simulink library "LibFactorGraph"  (Simulink 8.3)
settings: Solver=ode45  StartTime=0.0  StopTime=10.0  RelTol=1e-3
undefined symbols (not defined in the file or in its folder): bV, epsVal, eu, fcn, fP_0, fV, Hin_0, L_0, Nit_0, P_0, xi
libraries: LibFactorGraph x357
(part 2 of 4)

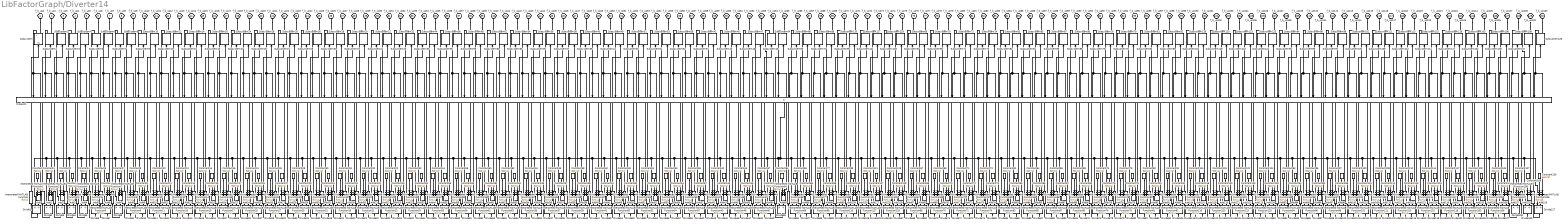
== system LibFactorGraph/Diverter14 ==
  Add{,1..129} (130 alike) : Sum
  Constant{,1..129} (130 alike) : Constant  Value=epsVal
  Divide{1..130} (130 alike) : Product  Inputs=*/
  Interpreted MATLAB Function{,1..129} (130 alike) : MATLABFcn  MATLABFcn=fcn(u)  Output1D=off
  Product1 : Product  Inputs=130  RndMeth=Zero
  Subsystem : Subsystem
  Subsystem{1..64,66..129} (128 alike) : LibFactorGraph/Diverter9/Subsystem
  Subsystem65 : LibFactorGraph/Diverter14/Subsystem
  f_b_up2 : PMIOPort  Port=1  Side=Left
  f_b_up1 : PMIOPort  Port=2  Side=Right
  f_b_up3 : PMIOPort  Port=3  Side=Left
  f_b_up4 : PMIOPort  Port=4  Side=Right
  f_b_up5 : PMIOPort  Port=5  Side=Left
  f_b_up6 : PMIOPort  Port=6  Side=Right
  f_b_up7 : PMIOPort  Port=7  Side=Left
  f_b_up8 : PMIOPort  Port=8  Side=Right
  f_b_up9 : PMIOPort  Port=9  Side=Left
  f_b_up10 : PMIOPort  Port=10  Side=Right
  f_b_up11 : PMIOPort  Port=11  Side=Left
  f_b_up12 : PMIOPort  Port=12  Side=Right
  f_b_up13 : PMIOPort  Port=13  Side=Left
  f_b_up14 : PMIOPort  Port=14  Side=Right
  f_b_up15 : PMIOPort  Port=15  Side=Left
  f_b_up16 : PMIOPort  Port=16  Side=Right
  f_b_up17 : PMIOPort  Port=17  Side=Left
  f_b_up18 : PMIOPort  Port=18  Side=Right
  f_b_up19 : PMIOPort  Port=19  Side=Left
  f_b_up20 : PMIOPort  Port=20  Side=Right
  f_b_up21 : PMIOPort  Port=21  Side=Left
  f_b_up22 : PMIOPort  Port=22  Side=Right
  f_b_up23 : PMIOPort  Port=23  Side=Left
  f_b_up24 : PMIOPort  Port=24  Side=Right
  f_b_up25 : PMIOPort  Port=25  Side=Left
  f_b_up26 : PMIOPort  Port=26  Side=Right
  f_b_up27 : PMIOPort  Port=27  Side=Left
  f_b_up28 : PMIOPort  Port=28  Side=Right
  f_b_up29 : PMIOPort  Port=29  Side=Left
  f_b_up30 : PMIOPort  Port=30  Side=Right
  f_b_up31 : PMIOPort  Port=31  Side=Left
  f_b_up32 : PMIOPort  Port=32  Side=Right
  f_b_up33 : PMIOPort  Port=33  Side=Left
  f_b_up34 : PMIOPort  Port=34  Side=Right
  f_b_up35 : PMIOPort  Port=35  Side=Left
  f_b_up36 : PMIOPort  Port=36  Side=Right
  f_b_up37 : PMIOPort  Port=37  Side=Left
  f_b_up38 : PMIOPort  Port=38  Side=Right
  f_b_up39 : PMIOPort  Port=39  Side=Left
  f_b_up40 : PMIOPort  Port=40  Side=Right
  f_b_up41 : PMIOPort  Port=41  Side=Left
  f_b_up42 : PMIOPort  Port=42  Side=Right
  f_b_up43 : PMIOPort  Port=43  Side=Left
  f_b_up44 : PMIOPort  Port=44  Side=Right
  f_b_up45 : PMIOPort  Port=45  Side=Left
  f_b_up46 : PMIOPort  Port=46  Side=Right
  f_b_up47 : PMIOPort  Port=47  Side=Left
  f_b_up48 : PMIOPort  Port=48  Side=Right
  f_b_up49 : PMIOPort  Port=49  Side=Left
  f_b_up50 : PMIOPort  Port=50  Side=Right
  f_b_up51 : PMIOPort  Port=51  Side=Left
  f_b_up52 : PMIOPort  Port=52  Side=Right
  f_b_up53 : PMIOPort  Port=53  Side=Left
  f_b_up54 : PMIOPort  Port=54  Side=Right
  f_b_up55 : PMIOPort  Port=55  Side=Left
  f_b_up56 : PMIOPort  Port=56  Side=Right
  f_b_up57 : PMIOPort  Port=57  Side=Left
  f_b_up58 : PMIOPort  Port=58  Side=Right
  f_b_up59 : PMIOPort  Port=59  Side=Left
  f_b_up60 : PMIOPort  Port=60  Side=Right
  f_b_up61 : PMIOPort  Port=61  Side=Left
  f_b_up62 : PMIOPort  Port=62  Side=Right
  f_b_up63 : PMIOPort  Port=63  Side=Left
  f_b_up64 : PMIOPort  Port=64  Side=Right
  f_b_up65 : PMIOPort  Port=65  Side=Left
  f_b_up66 : PMIOPort  Port=66  Side=Right
  f_b_up67 : PMIOPort  Port=67  Side=Left
  f_b_up68 : PMIOPort  Port=68  Side=Right
  f_b_up69 : PMIOPort  Port=69  Side=Left
  f_b_up70 : PMIOPort  Port=70  Side=Right
  f_b_up71 : PMIOPort  Port=71  Side=Left
  f_b_up72 : PMIOPort  Port=72  Side=Right
  f_b_up73 : PMIOPort  Port=73  Side=Left
  f_b_up74 : PMIOPort  Port=74  Side=Right
  f_b_up75 : PMIOPort  Port=75  Side=Left
  f_b_up76 : PMIOPort  Port=76  Side=Right
  f_b_up77 : PMIOPort  Port=77  Side=Left
  f_b_up78 : PMIOPort  Port=78  Side=Right
  f_b_up79 : PMIOPort  Port=79  Side=Left
  f_b_up80 : PMIOPort  Port=80  Side=Right
  f_b_up81 : PMIOPort  Port=81  Side=Left
  f_b_up82 : PMIOPort  Port=82  Side=Right
  f_b_up83 : PMIOPort  Port=83  Side=Left
  f_b_up84 : PMIOPort  Port=84  Side=Right
  f_b_up85 : PMIOPort  Port=85  Side=Left
  f_b_up86 : PMIOPort  Port=86  Side=Right
  f_b_up87 : PMIOPort  Port=87  Side=Left
  f_b_up88 : PMIOPort  Port=88  Side=Right
  f_b_up89 : PMIOPort  Port=89  Side=Left
  f_b_up90 : PMIOPort  Port=90  Side=Right
  f_b_up91 : PMIOPort  Port=91  Side=Left
  f_b_up92 : PMIOPort  Port=92  Side=Right
  f_b_up93 : PMIOPort  Port=93  Side=Left
  f_b_up94 : PMIOPort  Port=94  Side=Right
  f_b_up95 : PMIOPort  Port=95  Side=Left
  f_b_up96 : PMIOPort  Port=96  Side=Right
  f_b_up97 : PMIOPort  Port=97  Side=Left
  f_b_up98 : PMIOPort  Port=98  Side=Right
  f_b_up99 : PMIOPort  Port=99  Side=Left
  f_b_up100 : PMIOPort  Port=100  Side=Right
  f_b_up101 : PMIOPort  Port=101  Side=Left
  f_b_up102 : PMIOPort  Port=102  Side=Right
  f_b_up103 : PMIOPort  Port=103  Side=Left
  f_b_up104 : PMIOPort  Port=104  Side=Right
  f_b_up105 : PMIOPort  Port=105  Side=Left
  f_b_up106 : PMIOPort  Port=106  Side=Right
  f_b_up107 : PMIOPort  Port=107  Side=Left
  f_b_up108 : PMIOPort  Port=108  Side=Right
  f_b_up109 : PMIOPort  Port=109  Side=Left
  f_b_up110 : PMIOPort  Port=110  Side=Right
  f_b_up111 : PMIOPort  Port=111  Side=Left
  f_b_up112 : PMIOPort  Port=112  Side=Right
  f_b_up113 : PMIOPort  Port=113  Side=Left
  f_b_up114 : PMIOPort  Port=114  Side=Right
  f_b_up115 : PMIOPort  Port=115  Side=Left
  f_b_up116 : PMIOPort  Port=116  Side=Right
  f_b_up117 : PMIOPort  Port=117  Side=Left
  f_b_up118 : PMIOPort  Port=118  Side=Right
  f_b_up119 : PMIOPort  Port=119  Side=Left
  f_b_up120 : PMIOPort  Port=120  Side=Right
  f_b_up121 : PMIOPort  Port=121  Side=Left
  f_b_up122 : PMIOPort  Port=122  Side=Right
  f_b_up123 : PMIOPort  Port=123  Side=Left
  f_b_up124 : PMIOPort  Port=124  Side=Right
  f_b_up125 : PMIOPort  Port=125  Side=Left
  f_b_up126 : PMIOPort  Port=126  Side=Right
  f_b_up127 : PMIOPort  Port=127  Side=Left
  f_b_up128 : PMIOPort  Port=128  Side=Right
  f_b_up129 : PMIOPort  Port=129  Side=Left
  f_b_up130 : PMIOPort  Port=130  Side=Right
  wires:
  Constant/1 -> Add/1
  Interpreted MATLAB Function/1 -> Subsystem/1(In1)
  Subsystem/1(Out1) -> Product1/1, Add/2
  Divide1/1 -> Interpreted MATLAB Function/1
  Constant1/1 -> Add1/1
  Interpreted MATLAB Function1/1 -> Subsystem1/1
  Subsystem1/1 -> Product1/2, Add1/2
  Divide2/1 -> Interpreted MATLAB Function1/1
  Constant2/1 -> Add2/1
  Interpreted MATLAB Function2/1 -> Subsystem2/1
  Subsystem2/1 -> Product1/3, Add2/2
  Divide3/1 -> Interpreted MATLAB Function2/1
  Constant3/1 -> Add3/1
  Interpreted MATLAB Function3/1 -> Subsystem3/1
  Subsystem3/1 -> Product1/4, Add3/2
  Divide4/1 -> Interpreted MATLAB Function3/1
  Constant4/1 -> Add4/1
  Interpreted MATLAB Function4/1 -> Subsystem4/1
  Subsystem4/1 -> Product1/5, Add4/2
  Divide5/1 -> Interpreted MATLAB Function4/1
  Constant5/1 -> Add5/1
  Interpreted MATLAB Function5/1 -> Subsystem5/1
  Subsystem5/1 -> Product1/6, Add5/2
  Divide6/1 -> Interpreted MATLAB Function5/1
  Constant6/1 -> Add6/1
  Interpreted MATLAB Function6/1 -> Subsystem6/1
  Subsystem6/1 -> Product1/7, Add6/2
  Divide7/1 -> Interpreted MATLAB Function6/1
  Constant7/1 -> Add7/1
  Interpreted MATLAB Function7/1 -> Subsystem7/1
  Subsystem7/1 -> Product1/8, Add7/2
  Divide8/1 -> Interpreted MATLAB Function7/1
  Add/1 -> Divide1/2
  Add1/1 -> Divide2/2
  Add2/1 -> Divide3/2
  Add3/1 -> Divide4/2
  Add4/1 -> Divide5/2
  Add5/1 -> Divide6/2
  Add6/1 -> Divide7/2
  Add7/1 -> Divide8/2
  Constant8/1 -> Add8/1
  Interpreted MATLAB Function8/1 -> Subsystem8/1
  Subsystem8/1 -> Product1/9, Add8/2
  Divide9/1 -> Interpreted MATLAB Function8/1
  Constant9/1 -> Add9/1
  Interpreted MATLAB Function9/1 -> Subsystem9/1
  Subsystem9/1 -> Product1/10, Add9/2
  Divide10/1 -> Interpreted MATLAB Function9/1
  Constant10/1 -> Add10/1
  Interpreted MATLAB Function10/1 -> Subsystem10/1
  Subsystem10/1 -> Product1/11, Add10/2
  Divide11/1 -> Interpreted MATLAB Function10/1
  Constant11/1 -> Add11/1
  Interpreted MATLAB Function11/1 -> Subsystem11/1
  Subsystem11/1 -> Product1/12, Add11/2
  Divide12/1 -> Interpreted MATLAB Function11/1
  Constant12/1 -> Add12/1
  Interpreted MATLAB Function12/1 -> Subsystem12/1
  Subsystem12/1 -> Product1/13, Add12/2
  Divide13/1 -> Interpreted MATLAB Function12/1
  Constant13/1 -> Add13/1
  Interpreted MATLAB Function13/1 -> Subsystem13/1
  Subsystem13/1 -> Product1/14, Add13/2
  Divide14/1 -> Interpreted MATLAB Function13/1
  Constant14/1 -> Add14/1
  Interpreted MATLAB Function14/1 -> Subsystem14/1
  Subsystem14/1 -> Product1/15, Add14/2
  Divide15/1 -> Interpreted MATLAB Function14/1
  Constant15/1 -> Add15/1
  Interpreted MATLAB Function15/1 -> Subsystem15/1
  Subsystem15/1 -> Product1/16, Add15/2
  Divide16/1 -> Interpreted MATLAB Function15/1
  Add8/1 -> Divide9/2
  Add9/1 -> Divide10/2
  Add10/1 -> Divide11/2
  Add11/1 -> Divide12/2
  Add12/1 -> Divide13/2
  Add13/1 -> Divide14/2
  Add14/1 -> Divide15/2
  Add15/1 -> Divide16/2
  Constant16/1 -> Add16/1
  Interpreted MATLAB Function16/1 -> Subsystem16/1
  Subsystem16/1 -> Product1/17, Add16/2
  Divide17/1 -> Interpreted MATLAB Function16/1
  Constant17/1 -> Add17/1
  Interpreted MATLAB Function17/1 -> Subsystem17/1
  Subsystem17/1 -> Product1/18, Add17/2
  Divide25/1 -> Interpreted MATLAB Function17/1
  Constant24/1 -> Add24/1
  Interpreted MATLAB Function24/1 -> Subsystem24/1
  Subsystem24/1 -> Product1/19, Add24/2
  Divide26/1 -> Interpreted MATLAB Function24/1
  Constant25/1 -> Add25/1
  Interpreted MATLAB Function25/1 -> Subsystem25/1
  Subsystem25/1 -> Product1/20, Add25/2
  Divide27/1 -> Interpreted MATLAB Function25/1
  Constant26/1 -> Add26/1
  Interpreted MATLAB Function26/1 -> Subsystem26/1
  Subsystem26/1 -> Product1/21, Add26/2
  Divide28/1 -> Interpreted MATLAB Function26/1
  Constant27/1 -> Add27/1
  Interpreted MATLAB Function27/1 -> Subsystem27/1
  Subsystem27/1 -> Product1/22, Add27/2
  Divide29/1 -> Interpreted MATLAB Function27/1
  Constant28/1 -> Add28/1
  Interpreted MATLAB Function28/1 -> Subsystem28/1
  Subsystem28/1 -> Product1/23, Add28/2
  Divide30/1 -> Interpreted MATLAB Function28/1
  Constant29/1 -> Add29/1
  Interpreted MATLAB Function29/1 -> Subsystem29/1
  Subsystem29/1 -> Product1/24, Add29/2
  Divide31/1 -> Interpreted MATLAB Function29/1
  Add16/1 -> Divide17/2
  Add17/1 -> Divide25/2
  Add24/1 -> Divide26/2
  Add25/1 -> Divide27/2
  Add26/1 -> Divide28/2
  Add27/1 -> Divide29/2
  Add28/1 -> Divide30/2
  Add29/1 -> Divide31/2
  Constant30/1 -> Add30/1
  Interpreted MATLAB Function30/1 -> Subsystem30/1
  Subsystem30/1 -> Product1/25, Add30/2
  Divide32/1 -> Interpreted MATLAB Function30/1
  Constant31/1 -> Add31/1
  Interpreted MATLAB Function31/1 -> Subsystem31/1
  Subsystem31/1 -> Product1/26, Add31/2
  Divide18/1 -> Interpreted MATLAB Function31/1
  Constant18/1 -> Add18/1
  Interpreted MATLAB Function18/1 -> Subsystem18/1
  Subsystem18/1 -> Product1/27, Add18/2
  Divide19/1 -> Interpreted MATLAB Function18/1
  Constant19/1 -> Add19/1
  Interpreted MATLAB Function19/1 -> Subsystem19/1
  Subsystem19/1 -> Product1/28, Add19/2
  Divide20/1 -> Interpreted MATLAB Function19/1
  Constant20/1 -> Add20/1
  Interpreted MATLAB Function20/1 -> Subsystem20/1
  Subsystem20/1 -> Product1/29, Add20/2
  Divide21/1 -> Interpreted MATLAB Function20/1
  Constant21/1 -> Add21/1
  Interpreted MATLAB Function21/1 -> Subsystem21/1
  Subsystem21/1 -> Product1/30, Add21/2
  Divide22/1 -> Interpreted MATLAB Function21/1
  Constant22/1 -> Add22/1
  Interpreted MATLAB Function22/1 -> Subsystem22/1
  Subsystem22/1 -> Product1/31, Add22/2
  Divide23/1 -> Interpreted MATLAB Function22/1
  Constant23/1 -> Add23/1
  Interpreted MATLAB Function23/1 -> Subsystem23/1
  Subsystem23/1 -> Product1/32, Add23/2
  Divide24/1 -> Interpreted MATLAB Function23/1
  Add30/1 -> Divide32/2
  Add31/1 -> Divide18/2
  Add18/1 -> Divide19/2
  Add19/1 -> Divide20/2
  Add20/1 -> Divide21/2
  Add21/1 -> Divide22/2
  Add22/1 -> Divide23/2
  Add23/1 -> Divide24/2
  Constant32/1 -> Add32/1
  Interpreted MATLAB Function32/1 -> Subsystem32/1
  Subsystem32/1 -> Product1/33, Add32/2
  Divide33/1 -> Interpreted MATLAB Function32/1
  Constant33/1 -> Add33/1
  Interpreted MATLAB Function33/1 -> Subsystem33/1
  Subsystem33/1 -> Product1/34, Add33/2
  Divide44/1 -> Interpreted MATLAB Function33/1
  Constant44/1 -> Add44/1
  Interpreted MATLAB Function44/1 -> Subsystem44/1
  Subsystem44/1 -> Product1/35, Add44/2
  Divide55/1 -> Interpreted MATLAB Function44/1
  Constant55/1 -> Add55/1
  Interpreted MATLAB Function55/1 -> Subsystem55/1
  Subsystem55/1 -> Product1/36, Add55/2
  Divide59/1 -> Interpreted MATLAB Function55/1
  Constant58/1 -> Add58/1
  Interpreted MATLAB Function58/1 -> Subsystem58/1
  Subsystem58/1 -> Product1/37, Add58/2
  Divide60/1 -> Interpreted MATLAB Function58/1
  Constant59/1 -> Add59/1
  Interpreted MATLAB Function59/1 -> Subsystem59/1
  Subsystem59/1 -> Product1/38, Add59/2
  Divide61/1 -> Interpreted MATLAB Function59/1
  Constant60/1 -> Add60/1
  Interpreted MATLAB Function60/1 -> Subsystem60/1
  Subsystem60/1 -> Product1/39, Add60/2
  Divide62/1 -> Interpreted MATLAB Function60/1
  Constant61/1 -> Add61/1
  Interpreted MATLAB Function61/1 -> Subsystem61/1
  Subsystem61/1 -> Product1/40, Add61/2
  Divide63/1 -> Interpreted MATLAB Function61/1
  Add32/1 -> Divide33/2
  Add33/1 -> Divide44/2
  Add44/1 -> Divide55/2
  Add55/1 -> Divide59/2
  Add58/1 -> Divide60/2
  Add59/1 -> Divide61/2
  Add60/1 -> Divide62/2
  Add61/1 -> Divide63/2
  Constant62/1 -> Add62/1
  Interpreted MATLAB Function62/1 -> Subsystem62/1
  Subsystem62/1 -> Product1/41, Add62/2
  Divide64/1 -> Interpreted MATLAB Function62/1
  Constant63/1 -> Add63/1
  Interpreted MATLAB Function63/1 -> Subsystem63/1
  Subsystem63/1 -> Product1/42, Add63/2
  Divide34/1 -> Interpreted MATLAB Function63/1
  Constant34/1 -> Add34/1
  Interpreted MATLAB Function34/1 -> Subsystem34/1
  Subsystem34/1 -> Product1/43, Add34/2
  Divide35/1 -> Interpreted MATLAB Function34/1
  Constant35/1 -> Add35/1
  Interpreted MATLAB Function35/1 -> Subsystem35/1
  Subsystem35/1 -> Product1/44, Add35/2
  Divide36/1 -> Interpreted MATLAB Function35/1
  Constant36/1 -> Add36/1
  Interpreted MATLAB Function36/1 -> Subsystem36/1
  Subsystem36/1 -> Product1/45, Add36/2
  Divide37/1 -> Interpreted MATLAB Function36/1
  Constant37/1 -> Add37/1
  Interpreted MATLAB Function37/1 -> Subsystem37/1
  Subsystem37/1 -> Product1/46, Add37/2
  Divide38/1 -> Interpreted MATLAB Function37/1
  Constant38/1 -> Add38/1
  Interpreted MATLAB Function38/1 -> Subsystem38/1
  Subsystem38/1 -> Product1/47, Add38/2
  Divide39/1 -> Interpreted MATLAB Function38/1
  Constant39/1 -> Add39/1
  Interpreted MATLAB Function39/1 -> Subsystem39/1
  Subsystem39/1 -> Product1/48, Add39/2
  Divide40/1 -> Interpreted MATLAB Function39/1
  Add62/1 -> Divide64/2
  Add63/1 -> Divide34/2
  Add34/1 -> Divide35/2
  Add35/1 -> Divide36/2
  Add36/1 -> Divide37/2
  Add37/1 -> Divide38/2
  Add38/1 -> Divide39/2
  Add39/1 -> Divide40/2
  Constant40/1 -> Add40/1
  Interpreted MATLAB Function40/1 -> Subsystem40/1
  Subsystem40/1 -> Product1/49, Add40/2
  Divide41/1 -> Interpreted MATLAB Function40/1
  Constant41/1 -> Add41/1
  Interpreted MATLAB Function41/1 -> Subsystem41/1
  Subsystem41/1 -> Product1/50, Add41/2
  Divide50/1 -> Interpreted MATLAB Function41/1
  Constant49/1 -> Add49/1
  Interpreted MATLAB Function49/1 -> Subsystem49/1
  Subsystem49/1 -> Product1/51, Add49/2
  Divide51/1 -> Interpreted MATLAB Function49/1
  Constant50/1 -> Add50/1
  Interpreted MATLAB Function50/1 -> Subsystem50/1
  Subsystem50/1 -> Product1/52, Add50/2
  Divide52/1 -> Interpreted MATLAB Function50/1
  Constant51/1 -> Add51/1
  Interpreted MATLAB Function51/1 -> Subsystem51/1
  Subsystem51/1 -> Product1/53, Add51/2
  Divide53/1 -> Interpreted MATLAB Function51/1
  Constant52/1 -> Add52/1
  Interpreted MATLAB Function52/1 -> Subsystem52/1
  Subsystem52/1 -> Product1/54, Add52/2
  Divide54/1 -> Interpreted MATLAB Function52/1
  Constant53/1 -> Add53/1
  Interpreted MATLAB Function53/1 -> Subsystem53/1
  Subsystem53/1 -> Product1/55, Add53/2
  Divide56/1 -> Interpreted MATLAB Function53/1
  Constant54/1 -> Add54/1
  Interpreted MATLAB Function54/1 -> Subsystem54/1
  Subsystem54/1 -> Product1/56, Add54/2
  Divide57/1 -> Interpreted MATLAB Function54/1
  Add40/1 -> Divide41/2
  Add41/1 -> Divide50/2
  Add49/1 -> Divide51/2
  Add50/1 -> Divide52/2
  Add51/1 -> Divide53/2
  Add52/1 -> Divide54/2
  Add53/1 -> Divide56/2
  Add54/1 -> Divide57/2
  Constant56/1 -> Add56/1
  Interpreted MATLAB Function56/1 -> Subsystem56/1
  Subsystem56/1 -> Product1/57, Add56/2
  Divide58/1 -> Interpreted MATLAB Function56/1
  Constant57/1 -> Add57/1
  Interpreted MATLAB Function57/1 -> Subsystem57/1
  Subsystem57/1 -> Product1/58, Add57/2
  Divide42/1 -> Interpreted MATLAB Function57/1
  Constant42/1 -> Add42/1
  Interpreted MATLAB Function42/1 -> Subsystem42/1
  Subsystem42/1 -> Product1/59, Add42/2
  Divide43/1 -> Interpreted MATLAB Function42/1
  Constant43/1 -> Add43/1
  Interpreted MATLAB Function43/1 -> Subsystem43/1
  Subsystem43/1 -> Product1/60, Add43/2
  Divide45/1 -> Interpreted MATLAB Function43/1
  Constant45/1 -> Add45/1
  Interpreted MATLAB Function45/1 -> Subsystem45/1
  Subsystem45/1 -> Product1/61, Add45/2
  Divide46/1 -> Interpreted MATLAB Function45/1
  Constant46/1 -> Add46/1
  Interpreted MATLAB Function46/1 -> Subsystem46/1
  Subsystem46/1 -> Product1/62, Add46/2
  Divide47/1 -> Interpreted MATLAB Function46/1
  Constant47/1 -> Add47/1
  Interpreted MATLAB Function47/1 -> Subsystem47/1
  Subsystem47/1 -> Product1/63, Add47/2
  Divide48/1 -> Interpreted MATLAB Function47/1
  Interpreted MATLAB Function48/1 -> Subsystem48/1
  Subsystem48/1 -> Product1/64, Add64/2
  Divide49/1 -> Interpreted MATLAB Function48/1
  Add56/1 -> Divide58/2
  Add57/1 -> Divide42/2
  Add42/1 -> Divide43/2
  Add43/1 -> Divide45/2
  Add45/1 -> Divide46/2
  Add46/1 -> Divide47/2
  Add47/1 -> Divide48/2
  Add64/1 -> Divide49/2
  Constant64/1 -> Add65/1
  Interpreted MATLAB Function64/1 -> Subsystem64/1
  Subsystem64/1 -> Product1/65, Add65/2
  Divide65/1 -> Interpreted MATLAB Function64/1
  Add65/1 -> Divide65/2
  Constant48/1 -> Add64/1
  Constant65/1 -> Add48/1
  Interpreted MATLAB Function65/1 -> Subsystem65/1
  Subsystem65/1 -> Product1/66, Add48/2
  Divide66/1 -> Interpreted MATLAB Function65/1
  Product1/1 -> Divide127/1, Divide109/1, Divide108/1, Divide107/1, Divide106/1, Divide105/1, Divide103/1, Divide102/1, Divide119/1, Divide118/1, Divide117/1, Divide115/1, Divide114/1, Divide113/1, Divide112/1, Divide111/1, Divide101/1, Divide100/1, Divide98/1, Divide97/1, Divide96/1, Divide95/1, Divide94/1, Divide93/1, Divide126/1, Divide125/1, Divide124/1, Divide123/1, Divide122/1, Divide120/1, Divide116/1, Divide104/1, Divide92/1, Divide82/1, Divide81/1, Divide80/1, Divide79/1, Divide78/1, Divide76/1, Divide75/1, Divide91/1, Divide90/1, Divide89/1, Divide87/1, Divide86/1, Divide85/1, Divide84/1, Divide83/1, Divide74/1, Divide73/1, Divide72/1, Divide71/1, Divide70/1, Divide69/1, Divide68/1, Divide67/1, Divide130/1, Divide129/1, Divide128/1, Divide121/1, Divide110/1, Divide99/1, Divide88/1, Divide77/1, Divide66/1, Divide33/1, Divide24/1, Divide23/1, Divide22/1, Divide20/1, Divide19/1, Divide18/1, Divide32/1, Divide31/1, Divide30/1, Divide29/1, Divide28/1, Divide27/1, Divide26/1, Divide25/1, Divide17/1, Divide14/1, Divide13/1, Divide12/1, Divide10/1, Divide9/1, Divide8/1, Divide7/1, Divide6/1, Divide5/1, Divide4/1, Divide3/1, Divide2/1, Divide1/1, Divide11/1, Divide15/1, Divide16/1, Divide21/1, Divide44/1, Divide55/1, Divide59/1, Divide60/1, Divide61/1, Divide62/1, Divide63/1, Divide64/1, Divide34/1, Divide35/1, Divide36/1, Divide37/1, Divide38/1, Divide39/1, Divide40/1, Divide41/1, Divide50/1, Divide51/1, Divide52/1, Divide53/1, Divide54/1, Divide56/1, Divide57/1, Divide58/1, Divide42/1, Divide43/1, Divide45/1, Divide46/1, Divide47/1, Divide48/1, Divide49/1, Divide65/1
  Constant66/1 -> Add66/1
  Interpreted MATLAB Function66/1 -> Subsystem66/1
  Subsystem66/1 -> Product1/67, Add66/2
  Divide77/1 -> Interpreted MATLAB Function66/1
  Constant77/1 -> Add77/1
  Interpreted MATLAB Function77/1 -> Subsystem77/1
  Subsystem77/1 -> Product1/68, Add77/2
  Divide88/1 -> Interpreted MATLAB Function77/1
  Constant88/1 -> Add88/1
  Interpreted MATLAB Function88/1 -> Subsystem88/1
  Subsystem88/1 -> Product1/69, Add88/2
  Divide99/1 -> Interpreted MATLAB Function88/1
  Constant99/1 -> Add99/1
  Interpreted MATLAB Function99/1 -> Subsystem99/1
  Subsystem99/1 -> Product1/70, Add99/2
  Divide110/1 -> Interpreted MATLAB Function99/1
  Constant110/1 -> Add109/1
  Interpreted MATLAB Function110/1 -> Subsystem110/1
  Subsystem110/1 -> Product1/71, Add109/2
  Divide121/1 -> Interpreted MATLAB Function110/1
  Constant121/1 -> Add120/1
  Interpreted MATLAB Function121/1 -> Subsystem121/1
  Subsystem121/1 -> Product1/72, Add120/2
  Divide128/1 -> Interpreted MATLAB Function121/1
  Constant127/1 -> Add127/1
  Interpreted MATLAB Function127/1 -> Subsystem127/1
  Subsystem127/1 -> Product1/73, Add127/2
  Divide129/1 -> Interpreted MATLAB Function127/1
  Add48/1 -> Divide66/2
  Add66/1 -> Divide77/2
  Add77/1 -> Divide88/2
  Add88/1 -> Divide99/2
  Add99/1 -> Divide110/2
  Add109/1 -> Divide121/2
  Add120/1 -> Divide128/2
  Add127/1 -> Divide129/2
  Constant128/1 -> Add128/1
  Interpreted MATLAB Function128/1 -> Subsystem128/1
  Subsystem128/1 -> Product1/74, Add128/2
  Divide130/1 -> Interpreted MATLAB Function128/1
  Constant129/1 -> Add129/1
  Interpreted MATLAB Function129/1 -> Subsystem129/1
  Subsystem129/1 -> Product1/75, Add129/2
  Divide67/1 -> Interpreted MATLAB Function129/1
  Constant67/1 -> Add67/1
  Interpreted MATLAB Function67/1 -> Subsystem67/1
  Subsystem67/1 -> Product1/76, Add67/2
  Divide68/1 -> Interpreted MATLAB Function67/1
  Constant68/1 -> Add68/1
  Interpreted MATLAB Function68/1 -> Subsystem68/1
  Subsystem68/1 -> Product1/77, Add68/2
  Divide69/1 -> Interpreted MATLAB Function68/1
  Constant69/1 -> Add69/1
  Interpreted MATLAB Function69/1 -> Subsystem69/1
  Subsystem69/1 -> Product1/78, Add69/2
  Divide70/1 -> Interpreted MATLAB Function69/1
  Constant70/1 -> Add70/1
  Interpreted MATLAB Function70/1 -> Subsystem70/1
  Subsystem70/1 -> Product1/79, Add70/2
  Divide71/1 -> Interpreted MATLAB Function70/1
  Constant71/1 -> Add71/1
  Interpreted MATLAB Function71/1 -> Subsystem71/1
  Subsystem71/1 -> Product1/80, Add71/2
  Divide72/1 -> Interpreted MATLAB Function71/1
  Constant72/1 -> Add72/1
  Interpreted MATLAB Function72/1 -> Subsystem72/1
  Subsystem72/1 -> Product1/81, Add72/2
  Divide73/1 -> Interpreted MATLAB Function72/1
  Add128/1 -> Divide130/2
  Add129/1 -> Divide67/2
  Add67/1 -> Divide68/2
  Add68/1 -> Divide69/2
  Add69/1 -> Divide70/2
  Add70/1 -> Divide71/2
  Add71/1 -> Divide72/2
  Add72/1 -> Divide73/2
  Constant73/1 -> Add73/1
  Interpreted MATLAB Function73/1 -> Subsystem73/1
  Subsystem73/1 -> Product1/82, Add73/2
  Divide74/1 -> Interpreted MATLAB Function73/1
  Constant74/1 -> Add74/1
  Interpreted MATLAB Function74/1 -> Subsystem74/1
  Subsystem74/1 -> Product1/83, Add74/2
  Divide83/1 -> Interpreted MATLAB Function74/1
  Constant82/1 -> Add82/1
  Interpreted MATLAB Function82/1 -> Subsystem82/1
  Subsystem82/1 -> Product1/84, Add82/2
  Divide84/1 -> Interpreted MATLAB Function82/1
  Constant83/1 -> Add83/1
  Interpreted MATLAB Function83/1 -> Subsystem83/1
  Subsystem83/1 -> Product1/85, Add83/2
  Divide85/1 -> Interpreted MATLAB Function83/1
  Constant84/1 -> Add84/1
  Interpreted MATLAB Function84/1 -> Subsystem84/1
  Subsystem84/1 -> Product1/86, Add84/2
  Divide86/1 -> Interpreted MATLAB Function84/1
  Constant85/1 -> Add85/1
  Interpreted MATLAB Function85/1 -> Subsystem85/1
  Subsystem85/1 -> Product1/87, Add85/2
  Divide87/1 -> Interpreted MATLAB Function85/1
  Constant86/1 -> Add86/1
  Interpreted MATLAB Function86/1 -> Subsystem86/1
  Subsystem86/1 -> Product1/88, Add86/2
  Divide89/1 -> Interpreted MATLAB Function86/1
  Constant87/1 -> Add87/1
  Interpreted MATLAB Function87/1 -> Subsystem87/1
  Subsystem87/1 -> Product1/89, Add87/2
  Divide90/1 -> Interpreted MATLAB Function87/1
  Add73/1 -> Divide74/2
  Add74/1 -> Divide83/2
  Add82/1 -> Divide84/2
  Add83/1 -> Divide85/2
  Add84/1 -> Divide86/2
  Add85/1 -> Divide87/2
  Add86/1 -> Divide89/2
  Add87/1 -> Divide90/2
  Constant89/1 -> Add89/1
  Interpreted MATLAB Function89/1 -> Subsystem89/1
  Subsystem89/1 -> Product1/90, Add89/2
  Divide91/1 -> Interpreted MATLAB Function89/1
  Constant90/1 -> Add90/1
  Interpreted MATLAB Function90/1 -> Subsystem90/1
  Subsystem90/1 -> Product1/91, Add90/2
  Divide75/1 -> Interpreted MATLAB Function90/1
  Constant75/1 -> Add75/1
  Interpreted MATLAB Function75/1 -> Subsystem75/1
  Subsystem75/1 -> Product1/92, Add75/2
  Divide76/1 -> Interpreted MATLAB Function75/1
  Constant76/1 -> Add76/1
  Interpreted MATLAB Function76/1 -> Subsystem76/1
  Subsystem76/1 -> Product1/93, Add76/2
  Divide78/1 -> Interpreted MATLAB Function76/1
  Constant78/1 -> Add78/1
  Interpreted MATLAB Function78/1 -> Subsystem78/1
  Subsystem78/1 -> Product1/94, Add78/2
  Divide79/1 -> Interpreted MATLAB Function78/1
  Constant79/1 -> Add79/1
  Interpreted MATLAB Function79/1 -> Subsystem79/1
  Subsystem79/1 -> Product1/95, Add79/2
  Divide80/1 -> Interpreted MATLAB Function79/1
  Constant80/1 -> Add80/1
  Interpreted MATLAB Function80/1 -> Subsystem80/1
  Subsystem80/1 -> Product1/96, Add80/2
  Divide81/1 -> Interpreted MATLAB Function80/1
  Constant81/1 -> Add81/1
  Interpreted MATLAB Function81/1 -> Subsystem81/1
  Subsystem81/1 -> Product1/97, Add81/2
  Divide82/1 -> Interpreted MATLAB Function81/1
  Add89/1 -> Divide91/2
  Add90/1 -> Divide75/2
  Add75/1 -> Divide76/2
  Add76/1 -> Divide78/2
  Add78/1 -> Divide79/2
  Add79/1 -> Divide80/2
  Add80/1 -> Divide81/2
  Add81/1 -> Divide82/2
  Constant91/1 -> Add91/1
  Interpreted MATLAB Function91/1 -> Subsystem91/1
  Subsystem91/1 -> Product1/98, Add91/2
  Divide92/1 -> Interpreted MATLAB Function91/1
  Constant92/1 -> Add92/1
  Interpreted MATLAB Function92/1 -> Subsystem92/1
  Subsystem92/1 -> Product1/99, Add92/2
  Divide104/1 -> Interpreted MATLAB Function92/1
  Constant104/1 -> Add104/1
  Interpreted MATLAB Function104/1 -> Subsystem104/1
  Subsystem104/1 -> Product1/100, Add104/2
  Divide116/1 -> Interpreted MATLAB Function104/1
  Constant116/1 -> Add115/1
  Interpreted MATLAB Function116/1 -> Subsystem116/1
  Subsystem116/1 -> Product1/101, Add115/2
  Divide120/1 -> Interpreted MATLAB Function116/1
  Constant119/1 -> Add118/1
  Interpreted MATLAB Function119/1 -> Subsystem119/1
  Subsystem119/1 -> Product1/102, Add118/2
  Divide122/1 -> Interpreted MATLAB Function119/1
  Constant120/1 -> Add119/1
  Interpreted MATLAB Function120/1 -> Subsystem120/1
  Subsystem120/1 -> Product1/103, Add119/2
  Divide123/1 -> Interpreted MATLAB Function120/1
  Constant122/1 -> Add121/1
  Interpreted MATLAB Function122/1 -> Subsystem122/1
  Subsystem122/1 -> Product1/104, Add121/2
  Divide124/1 -> Interpreted MATLAB Function122/1
  Constant123/1 -> Add122/1
  Interpreted MATLAB Function123/1 -> Subsystem123/1
  Subsystem123/1 -> Product1/105, Add122/2
  Divide125/1 -> Interpreted MATLAB Function123/1
  Add91/1 -> Divide92/2
  Add92/1 -> Divide104/2
  Add104/1 -> Divide116/2
  Add115/1 -> Divide120/2
  Add118/1 -> Divide122/2
  Add119/1 -> Divide123/2
  Add121/1 -> Divide124/2
  Add122/1 -> Divide125/2
  Constant124/1 -> Add123/1
  Interpreted MATLAB Function124/1 -> Subsystem124/1
  Subsystem124/1 -> Product1/106, Add123/2
  Divide126/1 -> Interpreted MATLAB Function124/1
  Constant125/1 -> Add124/1
  Interpreted MATLAB Function125/1 -> Subsystem125/1
  Subsystem125/1 -> Product1/107, Add124/2
  Divide93/1 -> Interpreted MATLAB Function125/1
  Constant93/1 -> Add93/1
  Interpreted MATLAB Function93/1 -> Subsystem93/1
  Subsystem93/1 -> Product1/108, Add93/2
  Divide94/1 -> Interpreted MATLAB Function93/1
  Constant94/1 -> Add94/1
  Interpreted MATLAB Function94/1 -> Subsystem94/1
  Subsystem94/1 -> Product1/109, Add94/2
  Divide95/1 -> Interpreted MATLAB Function94/1
  Constant95/1 -> Add95/1
  Interpreted MATLAB Function95/1 -> Subsystem95/1
  Subsystem95/1 -> Product1/110, Add95/2
  Divide96/1 -> Interpreted MATLAB Function95/1
  Constant96/1 -> Add96/1
  Interpreted MATLAB Function96/1 -> Subsystem96/1
  Subsystem96/1 -> Product1/111, Add96/2
  Divide97/1 -> Interpreted MATLAB Function96/1
  Constant97/1 -> Add97/1
  Interpreted MATLAB Function97/1 -> Subsystem97/1
  Subsystem97/1 -> Product1/112, Add97/2
  Divide98/1 -> Interpreted MATLAB Function97/1
  Constant98/1 -> Add98/1
  Interpreted MATLAB Function98/1 -> Subsystem98/1
  Subsystem98/1 -> Product1/113, Add98/2
  Divide100/1 -> Interpreted MATLAB Function98/1
  Add123/1 -> Divide126/2
  Add124/1 -> Divide93/2
  Add93/1 -> Divide94/2
  Add94/1 -> Divide95/2
  Add95/1 -> Divide96/2
  Add96/1 -> Divide97/2
  Add97/1 -> Divide98/2
  Add98/1 -> Divide100/2
  Constant100/1 -> Add100/1
  Interpreted MATLAB Function100/1 -> Subsystem100/1
  Subsystem100/1 -> Product1/114, Add100/2
  Divide101/1 -> Interpreted MATLAB Function100/1
  Constant101/1 -> Add101/1
  Interpreted MATLAB Function101/1 -> Subsystem101/1
  Subsystem101/1 -> Product1/115, Add101/2
  Divide111/1 -> Interpreted MATLAB Function101/1
  Constant109/1 -> Add108/1
  Interpreted MATLAB Function109/1 -> Subsystem109/1
  Subsystem109/1 -> Product1/116, Add108/2
  Divide112/1 -> Interpreted MATLAB Function109/1
  Constant111/1 -> Add110/1
  Interpreted MATLAB Function111/1 -> Subsystem111/1
  Subsystem111/1 -> Product1/117, Add110/2
  Divide113/1 -> Interpreted MATLAB Function111/1
  Constant112/1 -> Add111/1
  Interpreted MATLAB Function112/1 -> Subsystem112/1
  Subsystem112/1 -> Product1/118, Add111/2
  Divide114/1 -> Interpreted MATLAB Function112/1
  Constant113/1 -> Add112/1
  Interpreted MATLAB Function113/1 -> Subsystem113/1
  Subsystem113/1 -> Product1/119, Add112/2
  Divide115/1 -> Interpreted MATLAB Function113/1
  Constant114/1 -> Add113/1
  Interpreted MATLAB Function114/1 -> Subsystem114/1
  Subsystem114/1 -> Product1/120, Add113/2
  Divide117/1 -> Interpreted MATLAB Function114/1
  Constant115/1 -> Add114/1
  Interpreted MATLAB Function115/1 -> Subsystem115/1
  Subsystem115/1 -> Product1/121, Add114/2
  Divide118/1 -> Interpreted MATLAB Function115/1
  Add100/1 -> Divide101/2
  Add101/1 -> Divide111/2
  Add108/1 -> Divide112/2
  Add110/1 -> Divide113/2
  Add111/1 -> Divide114/2
  Add112/1 -> Divide115/2
  Add113/1 -> Divide117/2
  Add114/1 -> Divide118/2
  Constant117/1 -> Add116/1
  Interpreted MATLAB Function117/1 -> Subsystem117/1
  Subsystem117/1 -> Product1/122, Add116/2
  Divide119/1 -> Interpreted MATLAB Function117/1
  Constant118/1 -> Add117/1
  Interpreted MATLAB Function118/1 -> Subsystem118/1
  Subsystem118/1 -> Product1/123, Add117/2
  Divide102/1 -> Interpreted MATLAB Function118/1
  Constant102/1 -> Add102/1
  Interpreted MATLAB Function102/1 -> Subsystem102/1
  Subsystem102/1 -> Product1/124, Add102/2
  Divide103/1 -> Interpreted MATLAB Function102/1
  Constant103/1 -> Add103/1
  Interpreted MATLAB Function103/1 -> Subsystem103/1
  Subsystem103/1 -> Product1/125, Add103/2
  Divide105/1 -> Interpreted MATLAB Function103/1
  Constant105/1 -> Add105/1
  Interpreted MATLAB Function105/1 -> Subsystem105/1
  Subsystem105/1 -> Product1/126, Add105/2
  Divide106/1 -> Interpreted MATLAB Function105/1
  Constant106/1 -> Add106/1
  Interpreted MATLAB Function106/1 -> Subsystem106/1
  Subsystem106/1 -> Product1/127, Add106/2
  Divide107/1 -> Interpreted MATLAB Function106/1
  Constant107/1 -> Add107/1
  Interpreted MATLAB Function107/1 -> Subsystem107/1
  Subsystem107/1 -> Product1/128, Add107/2
  Divide108/1 -> Interpreted MATLAB Function107/1
  Interpreted MATLAB Function108/1 -> Subsystem108/1
  Subsystem108/1 -> Product1/129, Add125/2
  Divide109/1 -> Interpreted MATLAB Function108/1
  Add116/1 -> Divide119/2
  Add117/1 -> Divide102/2
  Add102/1 -> Divide103/2
  Add103/1 -> Divide105/2
  Add105/1 -> Divide106/2
  Add106/1 -> Divide107/2
  Add107/1 -> Divide108/2
  Add125/1 -> Divide109/2
  Constant126/1 -> Add126/1
  Interpreted MATLAB Function126/1 -> Subsystem126/1
  Subsystem126/1 -> Product1/130, Add126/2
  Divide127/1 -> Interpreted MATLAB Function126/1
  Add126/1 -> Divide127/2
  Constant108/1 -> Add125/1
  connections:
  f_b_up2/RConn1 -- Subsystem/RConn1
  f_b_up1/RConn1 -- Subsystem1/RConn1
  f_b_up4/RConn1 -- Subsystem3/RConn1
  f_b_up3/RConn1 -- Subsystem2/RConn1
  f_b_up5/RConn1 -- Subsystem4/RConn1
  f_b_up6/RConn1 -- Subsystem5/RConn1
  f_b_up8/RConn1 -- Subsystem7/RConn1
  f_b_up7/RConn1 -- Subsystem6/RConn1
  f_b_up9/RConn1 -- Subsystem8/RConn1
  f_b_up10/RConn1 -- Subsystem9/RConn1
  f_b_up15/RConn1 -- Subsystem14/RConn1
  f_b_up16/RConn1 -- Subsystem15/RConn1
  f_b_up11/RConn1 -- Subsystem10/RConn1
  f_b_up12/RConn1 -- Subsystem11/RConn1
  f_b_up13/RConn1 -- Subsystem12/RConn1
  f_b_up14/RConn1 -- Subsystem13/RConn1
  f_b_up27/RConn1 -- Subsystem18/RConn1
  f_b_up28/RConn1 -- Subsystem19/RConn1
  f_b_up25/RConn1 -- Subsystem30/RConn1
  f_b_up20/RConn1 -- Subsystem25/RConn1
  f_b_up30/RConn1 -- Subsystem21/RConn1
  f_b_up24/RConn1 -- Subsystem29/RConn1
  f_b_up29/RConn1 -- Subsystem20/RConn1
  f_b_up26/RConn1 -- Subsystem31/RConn1
  f_b_up23/RConn1 -- Subsystem28/RConn1
  f_b_up22/RConn1 -- Subsystem27/RConn1
  f_b_up18/RConn1 -- Subsystem17/RConn1
  f_b_up21/RConn1 -- Subsystem26/RConn1
  f_b_up32/RConn1 -- Subsystem23/RConn1
  f_b_up31/RConn1 -- Subsystem22/RConn1
  f_b_up19/RConn1 -- Subsystem24/RConn1
  f_b_up17/RConn1 -- Subsystem16/RConn1
  f_b_up34/RConn1 -- Subsystem33/RConn1
  f_b_up37/RConn1 -- Subsystem58/RConn1
  f_b_up38/RConn1 -- Subsystem59/RConn1
  f_b_up39/RConn1 -- Subsystem60/RConn1
  f_b_up51/RConn1 -- Subsystem49/RConn1
  f_b_up47/RConn1 -- Subsystem38/RConn1
  f_b_up35/RConn1 -- Subsystem44/RConn1
  f_b_up36/RConn1 -- Subsystem55/RConn1
  f_b_up46/RConn1 -- Subsystem37/RConn1
  f_b_up33/RConn1 -- Subsystem32/RConn1
  f_b_up55/RConn1 -- Subsystem53/RConn1
  f_b_up48/RConn1 -- Subsystem39/RConn1
  f_b_up62/RConn1 -- Subsystem46/RConn1
  f_b_up42/RConn1 -- Subsystem63/RConn1
  f_b_up54/RConn1 -- Subsystem52/RConn1
  f_b_up58/RConn1 -- Subsystem57/RConn1
  f_b_up56/RConn1 -- Subsystem54/RConn1
  f_b_up43/RConn1 -- Subsystem34/RConn1
  f_b_up59/RConn1 -- Subsystem42/RConn1
  f_b_up45/RConn1 -- Subsystem36/RConn1
  f_b_up44/RConn1 -- Subsystem35/RConn1
  f_b_up41/RConn1 -- Subsystem62/RConn1
  f_b_up57/RConn1 -- Subsystem56/RConn1
  f_b_up53/RConn1 -- Subsystem51/RConn1
  f_b_up63/RConn1 -- Subsystem47/RConn1
  f_b_up61/RConn1 -- Subsystem45/RConn1
  f_b_up52/RConn1 -- Subsystem50/RConn1
  f_b_up40/RConn1 -- Subsystem61/RConn1
  f_b_up60/RConn1 -- Subsystem43/RConn1
  f_b_up49/RConn1 -- Subsystem40/RConn1
  f_b_up50/RConn1 -- Subsystem41/RConn1
  f_b_up64/RConn1 -- Subsystem48/RConn1
  f_b_up65/RConn1 -- Subsystem64/RConn1
  f_b_up99/RConn1 -- Subsystem92/RConn1
  f_b_up82/RConn1 -- Subsystem73/RConn1
  f_b_up103/RConn1 -- Subsystem120/RConn1
  f_b_up102/RConn1 -- Subsystem119/RConn1
  f_b_up107/RConn1 -- Subsystem125/RConn1
  f_b_up127/RConn1 -- Subsystem106/RConn1
  f_b_up90/RConn1 -- Subsystem89/RConn1
  f_b_up93/RConn1 -- Subsystem76/RConn1
  f_b_up88/RConn1 -- Subsystem86/RConn1
  f_b_up91/RConn1 -- Subsystem90/RConn1
  f_b_up67/RConn1 -- Subsystem66/RConn1
  f_b_up66/RConn1 -- Subsystem65/RConn1
  f_b_up68/RConn1 -- Subsystem77/RConn1
  f_b_up69/RConn1 -- Subsystem88/RConn1
  f_b_up75/RConn1 -- Subsystem129/RConn1
  f_b_up74/RConn1 -- Subsystem128/RConn1
  f_b_up94/RConn1 -- Subsystem78/RConn1
  f_b_up89/RConn1 -- Subsystem87/RConn1
  f_b_up95/RConn1 -- Subsystem79/RConn1
  f_b_up85/RConn1 -- Subsystem83/RConn1
  f_b_up124/RConn1 -- Subsystem102/RConn1
  f_b_up108/RConn1 -- Subsystem93/RConn1
  f_b_up121/RConn1 -- Subsystem115/RConn1
  f_b_up112/RConn1 -- Subsystem97/RConn1
  f_b_up98/RConn1 -- Subsystem91/RConn1
  f_b_up111/RConn1 -- Subsystem96/RConn1
  f_b_up128/RConn1 -- Subsystem107/RConn1
  f_b_up118/RConn1 -- Subsystem112/RConn1
  f_b_up122/RConn1 -- Subsystem117/RConn1
  f_b_up106/RConn1 -- Subsystem124/RConn1
  f_b_up113/RConn1 -- Subsystem98/RConn1
  f_b_up120/RConn1 -- Subsystem114/RConn1
  f_b_up72/RConn1 -- Subsystem121/RConn1
  f_b_up73/RConn1 -- Subsystem127/RConn1
  f_b_up130/RConn1 -- Subsystem126/RConn1
  f_b_up115/RConn1 -- Subsystem101/RConn1
  f_b_up114/RConn1 -- Subsystem100/RConn1
  f_b_up109/RConn1 -- Subsystem94/RConn1
  f_b_up110/RConn1 -- Subsystem95/RConn1
  f_b_up97/RConn1 -- Subsystem81/RConn1
  f_b_up86/RConn1 -- Subsystem84/RConn1
  f_b_up84/RConn1 -- Subsystem82/RConn1
  f_b_up96/RConn1 -- Subsystem80/RConn1
  f_b_up116/RConn1 -- Subsystem109/RConn1
  f_b_up104/RConn1 -- Subsystem122/RConn1
  f_b_up117/RConn1 -- Subsystem111/RConn1
  f_b_up126/RConn1 -- Subsystem105/RConn1
  f_b_up123/RConn1 -- Subsystem118/RConn1
  f_b_up119/RConn1 -- Subsystem113/RConn1
  f_b_up129/RConn1 -- Subsystem108/RConn1
  f_b_up83/RConn1 -- Subsystem74/RConn1
  f_b_up87/RConn1 -- Subsystem85/RConn1
  f_b_up101/RConn1 -- Subsystem116/RConn1
  f_b_up100/RConn1 -- Subsystem104/RConn1
  f_b_up125/RConn1 -- Subsystem103/RConn1
  f_b_up105/RConn1 -- Subsystem123/RConn1
  f_b_up76/RConn1 -- Subsystem67/RConn1
  f_b_up81/RConn1 -- Subsystem72/RConn1
  f_b_up80/RConn1 -- Subsystem71/RConn1
  f_b_up71/RConn1 -- Subsystem110/RConn1
  f_b_up70/RConn1 -- Subsystem99/RConn1
  f_b_up92/RConn1 -- Subsystem75/RConn1
  f_b_up79/RConn1 -- Subsystem70/RConn1
  f_b_up78/RConn1 -- Subsystem69/RConn1
  f_b_up77/RConn1 -- Subsystem68/RConn1
